simulink model "CLA_Sample"  (R2022b)
settings: Solver=FixedStepAuto  StartTime=0.0  StopTime=Inf  RelTol=1e-3  EnableMultiTasking=on
model workspace (MAT data in the model file):
  ADC_Gain = 1241.21212121
  DAC_Gain = 0.000805860805861
  Inductor_Current_Divider_Gain_Phase_A = 33.4
  Inductor_Current_Divider_Gain_Phase_B = 33.4
  Vbulk_Divider_Gain = 276.854928018
  Vin_Divider_Gain = 556.17352614
undefined symbols (not defined in the file or in its folder): GPTRIP1SEL, GPTRIP2SEL, SCI_A_Transmit, SCI_A_Transmit_Current_Suffix, SCI_A_Transmit_one_shot_Suffix, SCI_A_Transmit_Polarity_Suffix, SCI_A_Transmit_relay_Suffix, SCI_A_Transmit_Vbulk_Suffix, SCI_A_Transmit_Vin_rms_Suffix, SCI_A_Transmit_Vin_Suffix, SCI_A_Transmit_Vmid_Suffix, SCI_A_Transmit_Vp_Suffix, SCI_A_Transmit_Vpfc_Suffix, TZ1, TZ2
libraries: c280xlib x33, simulink x17, c2802xlib x15, c2000lib x1, c2806xlib x1
(part 2 of 5)

== system CLA_Sample/Calibration,RMS, Fault Protection @5kHz/Relay control ==
  note: 0.2 x ms
  note: This block will be executed at every 1 mili second. (1kHz)
  function : TriggerPort  TriggerType=function-call  VariantControl=(inherit)
  ADC Gain : Subsystem
  Data Store Memory1 : DataStoreMemory  DataStoreName=RELAY_START_DELAY  WriteAfterWriteMsg=warning  ShowAdditionalParam=off
  Data Store Read1 : DataStoreRead  DataStoreName=RELAY_START_DELAY  IndexOptions=Index vector (dialog)  Indices=1  OutputSizes=1
  Data Store Read3 : DataStoreRead  DataStoreName=Vin_peak_ADC_Phase_A  IndexOptions=Index vector (dialog)  Indices=1  OutputSizes=1
  Data Store Read4 : DataStoreRead  DataStoreName=Relay_TurnON_Threshold  IndexOptions=Index vector (dialog)  Indices=1  OutputSizes=1
  Data Store Read5 : DataStoreRead  DataStoreName=PFC_en  IndexOptions=Index vector (dialog)  Indices=1  OutputSizes=1
  Data Store Write1 : DataStoreWrite  DataStoreName=RELAY_START_DELAY  IndexOptions=Index vector (dialog)  Indices=1  OutputSizes=1
  Data Store Write6 : DataStoreWrite  DataStoreName=Relay_started  IndexOptions=Index vector (dialog)  Indices=1  OutputSizes=1
  Relay_Control : Stateflow chart  TreatAsAtomicUnit=on
  Relay_GPIO1 : c280xlib/Digital Output  GPIO_Number=GPIO8~GPIO15  GPIO_Bit0=on  GPIO_BIT0_Toggle=off  GPIO_Bit1=off  GPIO_BIT1_Toggle=off  GPIO_Bit2=off  GPIO_BIT2_Toggle=off  GPIO_Bit3=off  GPIO_BIT3_Toggle=off  GPIO_Bit4=off  GPIO_BIT4_Toggle=off  GPIO_Bit5=off  GPIO_BIT5_Toggle=off  GPIO_Bit6=off  GPIO_BIT6_Toggle=off  GPIO_Bit7=off  GPIO_BIT7_Toggle=off
  Subsystem : Subsystem  Commented=on
  ms : Constant  Value=150
  wires:
  ADC Gain/1(Out1) -> Relay_Control/2(Relay_TurnON_Threshold_ADC)
  Data Store Read5/1 -> Relay_Control/4(PFC_en)
  ms/1 -> Data Store Write1/1
  Relay_Control/2(PWM_Turned_on) -> Data Store Write6/1
  Data Store Read4/1 -> ADC Gain/1(In1)
  Relay_Control/1(Relay_Started) -> Relay_GPIO1/1
  Data Store Read1/1 -> Relay_Control/3(RELAY_START_DELAY)
  Data Store Read3/1 -> Relay_Control/1(Vin_peak_ADC)

== system CLA_Sample/Calibration,RMS, Fault Protection @5kHz/Soft Start ==
  note: This will be used for control computation.
  function : TriggerPort  TriggerType=function-call  VariantControl=(inherit)
  Chart : Stateflow chart  TreatAsAtomicUnit=on
      settings: PortSchema="{\"entries\":[{\"content\":{\"sides\":[{\"content\":{\"connectorIds\":[\"In2\",\"In3\",\"In4\",\"In5\",\"In6\"]},\"type\":\"ConnectorPlacement.EquallySpacedRectSide\",\"uuid\":\"22b210d6-ceb6-4123-9311-ecfc1554a514\"},{\"content\":{\"connectorIds\":[\"Out2\",\"Out3\",\"Out4\"],\"side\":\"RIGHT\"},\"type\":\"ConnectorPlacement.EquallySpacedRectSide\",\"uuid\":\"bd71c4d7-1c84-49a9-97ae-3dc5e1ac2530\"},{\"content\":{\"connectorIds\":[\"In1\",\"Out1\"],\"side\":\"TOP\"},\"type\":\"ConnectorPlacement.EquallySpacedRectSide\",\"uuid\":\"720c9beb-f716-4abe-bf9b-a08f9ee3742e\"}]},\"type\":\"ConnectorPlacement.EquallySpacedConnector\",\"uuid\":\"ea96fba9-9c4e-4b61-9de0-918baa6c198f\"}],\"packageUris\":[\"http://schema.mathworks.com/mf0/Connector/R2020b\"],\"version\":\"1.0\"}"
  Data Store Read : DataStoreRead  DataStoreName=Relay_started  IndexOptions=Index vector (dialog)  Indices=1  OutputSizes=1
  Data Store Read1 : DataStoreRead  DataStoreName=Vbulk_ADC  IndexOptions=Index vector (dialog)  Indices=1  OutputSizes=1
  Data Store Read2 : DataStoreRead  DataStoreName=First_Pass  IndexOptions=Index vector (dialog)  Indices=1  OutputSizes=1
  Data Store Read3 : DataStoreRead  DataStoreName=Soft_Start  IndexOptions=Index vector (dialog)  Indices=1  OutputSizes=1
  Data Store Read4 : DataStoreRead  DataStoreName=Vbulk_Ref_ADC  IndexOptions=Index vector (dialog)  Indices=1  OutputSizes=1
  Data Store Read5 : DataStoreRead  DataStoreName=PFC_en  IndexOptions=Index vector (dialog)  Indices=1  OutputSizes=1
  Data Store Write : DataStoreWrite  DataStoreName=First_Pass  IndexOptions=Index vector (dialog)  Indices=1  OutputSizes=1
  Data Store Write2 : DataStoreWrite  DataStoreName=Vbulk_Ref_ADC_adjusted  IndexOptions=Index vector (dialog)  Indices=1  OutputSizes=1
  Data Store Write3 : DataStoreWrite  DataStoreName=Soft_Start  IndexOptions=Index vector (dialog)  Indices=1  OutputSizes=1
  wires:
  Data Store Read1/1 -> Chart/3(Vbulk_ADC)
  Data Store Read2/1 -> Chart/4("First_Pass ")
  Chart/2(First_Pass) -> Data Store Write/1
  Data Store Read3/1 -> Chart/5("Soft_Start ")
  Data Store Read4/1 -> Chart/6(Vbulk_Ref_ADC)
  Chart/4(Vbulk_Ref_ADC_adjusted) -> Data Store Write2/1
  Chart/3(Soft_Start) -> Data Store Write3/1
  Data Store Read5/1 -> Chart/2(PFC_en)
  Data Store Read/1 -> Chart/1(Relay_started)

== system CLA_Sample/Calibration,RMS, Fault Protection @5kHz/Voltage RMS//Averag Calculation ==
  function : TriggerPort  TriggerType=function-call  VariantControl=(inherit)
  Function-Call Generator : simulink/Ports & Subsystems/Function-Call Generator  sample_time=-1  numberOfIterations=1  DisallowWideOutput=off
  Function-Call Split : FunctionCallSplit  IconShape=distinctive  NumOutputPorts=4  OutputPortLayout=default
  Phase_A : Subsystem  TreatAsAtomicUnit=on
  Phase_B : Subsystem  TreatAsAtomicUnit=on
  Phase_C : Subsystem  TreatAsAtomicUnit=on
  Vbulk_ADC Averaging : Subsystem  TreatAsAtomicUnit=on
  wires:
  Function-Call Generator/1 -> Function-Call Split/1
  Function-Call Split/1 -> Vbulk_ADC Averaging/Trigger
  Function-Call Split/2 -> Phase_A/Trigger
  Function-Call Split/3 -> Phase_B/Trigger
  Function-Call Split/4 -> Phase_C/Trigger

== system CLA_Sample/Duty update via UART/Simulink Function ==
  note: Ascii to number
  SCI_Receive : TriggerPort  TriggerType=function-call  IsSimulinkFunction=on  FunctionName=SCI_Receive  FunctionVisibility=scoped  VariantControl=(inherit)
  Constant2 : Constant  Value=48
  Constant3 : Constant  Value=48
  Constant4 : Constant  Value=48
  Demux : Demux  Outputs=3
  Gain2 : Gain  Gain=100
  Gain3 : Gain  Gain=10
  Gain4 : Gain
  SCI Receive : c280xlib/SCI Receive  Priority=2  sciModule=A  dataHead=''  headerCheckMaxCount=16  dataTail=''  dataType=uint8  dataLenOptions=Length via dialog  dataDim=3  maxDataLength=100  initValue=0  errOption=Output custom value  errValue=0  sampleTime=-1  blockingMode=on  timeOut=0.01944  outputStatus=off
      settings: LibrarySourceBlock=c2806xlib/SCI Receive
  Sum2 : Sum  Inputs=|+-
  Sum3 : Sum  Inputs=|+-
  Sum4 : Sum  Inputs=|+-
  Sum5 : Sum  Inputs=|+++  AccumDataTypeStr=double  OutDataTypeStr=double
  y : ArgOut  DisableCoverage=on  ArgumentName=y
  wires:
  Constant4/1 -> Sum4/2
  SCI Receive/1 -> Demux/1
  Gain4/1 -> Sum5/3
  Constant2/1 -> Sum2/2
  Demux/1 -> Sum2/1
  Sum3/1 -> Gain3/1
  Demux/2 -> Sum3/1
  Demux/3 -> Sum4/1
  Sum4/1 -> Gain4/1
  Constant3/1 -> Sum3/2
  Sum2/1 -> Gain2/1
  Gain2/1 -> Sum5/1
  Gain3/1 -> Sum5/2
  Sum5/1 -> y/1

== system CLA_Sample/Initialize Function/Subsystem1 ==
  kHz : Inport
  % : Inport  Port=2
  Constant1 : Constant  Value=90E6
  Constant2 : Constant
  Divide : Product  Inputs=*/  RndMeth=Zero  SaturateOnIntegerOverflow=on
  Gain : Gain  Gain=1000
  Gain1 : Gain  Gain=1/100
  Product1 : Product
  Subtract : Sum  Inputs=+-
  Out1 : Outport
  Out2 : Outport  Port=2
  wires:
  kHz/1 -> Gain/1
  Constant1/1 -> Divide/1
  Gain/1 -> Divide/2
  Divide/1 -> Product1/1, Out1/1
  %/1 -> Gain1/1
  Constant2/1 -> Subtract/1
  Gain1/1 -> Subtract/2
  Subtract/1 -> Product1/2
  Product1/1 -> Out2/1

== system CLA_Sample/Initialize Function/Subsystem2 ==
  Hz : Inport
  Duty : Inport  Port=2
  128*14 divider : Gain  Gain=1/(128*14)
  Constant1 : Constant  Value=90E6
  Constant2 : Constant
  Divide : Product  Inputs=*/  RndMeth=Zero  SaturateOnIntegerOverflow=on
  Floor : Rounding  Operator=round
  Floor1 : Rounding  Operator=round
  Gain1 : Gain  Gain=1/100
  Product1 : Product
  Subtract : Sum  Inputs=+-
  Out1 : Outport
  Out2 : Outport  Port=2
  wires:
  Duty/1 -> Gain1/1
  Divide/1 -> Floor/1, Product1/1
  Floor1/1 -> Out2/1
  Hz/1 -> 128*14 divider/1
  128*14 divider/1 -> Divide/2
  Constant2/1 -> Subtract/1
  Gain1/1 -> Subtract/2
  Constant1/1 -> Divide/1
  Subtract/1 -> Product1/2
  Product1/1 -> Floor1/1
  Floor/1 -> Out1/1

== system CLA_Sample/Initialize Function/Subsystem3 ==
  kHz : Inport
  % : Inport  Port=2
  Constant1 : Constant  Value=90E6
  Constant2 : Constant
  Divide : Product  Inputs=*/  RndMeth=Zero  SaturateOnIntegerOverflow=on
  Gain : Gain  Gain=1000
  Gain1 : Gain  Gain=1/100
  Product1 : Product
  Subtract : Sum  Inputs=+-
  Out1 : Outport
  Out2 : Outport  Port=2
  wires:
  kHz/1 -> Gain/1
  Constant1/1 -> Divide/1
  Gain/1 -> Divide/2
  Divide/1 -> Product1/1, Out1/1
  %/1 -> Gain1/1
  Constant2/1 -> Subtract/1
  Gain1/1 -> Subtract/2
  Subtract/1 -> Product1/2
  Product1/1 -> Out2/1

== system CLA_Sample/PWM Update @65KHz/Closed loop PWM generation (Control) ==
  function : TriggerPort  TriggerType=function-call  VariantControl=(inherit)
  Data Store Read1 : DataStoreRead  DataStoreName=Relay_started  IndexOptions=Index vector (dialog)  Indices=1  OutputSizes=1
  Data Store Read7 : DataStoreRead  DataStoreName=PFC_en  IndexOptions=Index vector (dialog)  Indices=1  OutputSizes=1
  If : If  NumInputs=2  IfExpression=(u1 ==1) & (u2==1)  ShowElse=off
  If Action Subsystem : Subsystem  TreatAsAtomicUnit=on
  wires:
  Data Store Read7/1 -> If/1
  If/1 -> If Action Subsystem/Action
  Data Store Read1/1 -> If/2

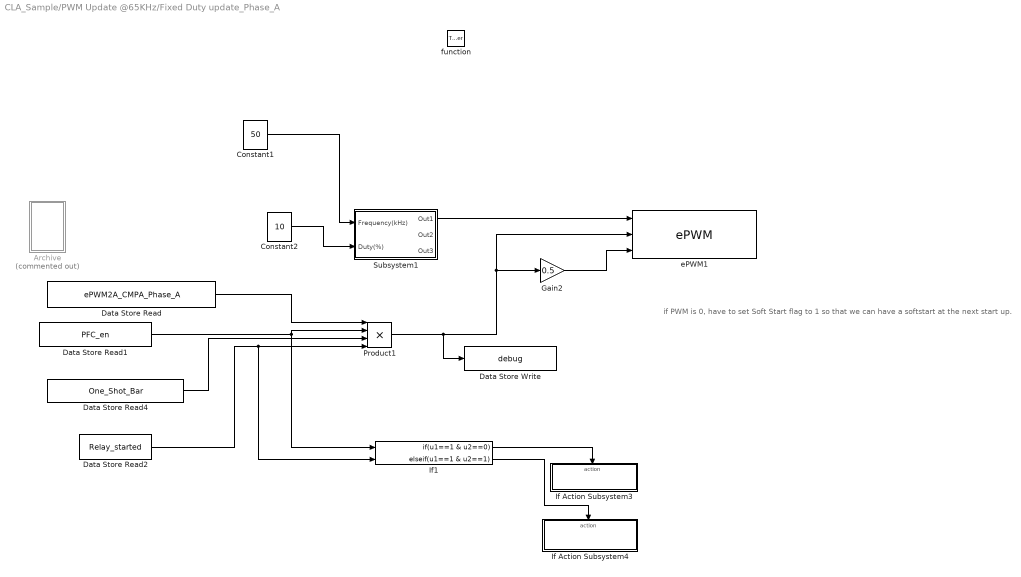
== system CLA_Sample/PWM Update @65KHz/Fixed Duty update_Phase_A ==
  note: if PWM is 0, have to set Soft Start flag to 1 so that we can have a softstart at the next start up.
  function : TriggerPort  TriggerType=function-call  VariantControl=(inherit)
  Archive : Subsystem  Commented=on
  Constant1 : Constant  Value=50
  Constant2 : Constant  Value=10
  Data Store Read : DataStoreRead  DataStoreName=ePWM2A_CMPA_Phase_A  IndexOptions=Index vector (dialog)  Indices=1  OutputSizes=1
  Data Store Read1 : DataStoreRead  DataStoreName=PFC_en  IndexOptions=Index vector (dialog)  Indices=1  OutputSizes=1
  Data Store Read2 : DataStoreRead  DataStoreName=Relay_started  IndexOptions=Index vector (dialog)  Indices=1  OutputSizes=1
  Data Store Read4 : DataStoreRead  DataStoreName=One_Shot_Bar  IndexOptions=Index vector (dialog)  Indices=1  OutputSizes=1
  Data Store Write : DataStoreWrite  DataStoreName=debug  IndexOptions=Index vector (dialog)  Indices=1  OutputSizes=1
  Gain2 : Gain  Gain=0.5
  If Action Subsystem3 : Subsystem  TreatAsAtomicUnit=on
  If Action Subsystem4 : Subsystem  TreatAsAtomicUnit=on
  If1 : If  NumInputs=2  IfExpression=u1==1 & u2==0  ElseIfExpressions=u1==1 & u2==1  ShowElse=off
  Product1 : Product  Inputs=4  OutDataTypeStr=double
  Subsystem1 : Subsystem
  ePWM1 : c2802xlib/ePWM  PwmType=C2000  useModule=ePWM2  ePWMxLINKTBPRD=Not Linked  periodUnits=Clock cycles  timerSource=Input port  timerPeriod_clk=1384  timerPeriod_sec=0.0001  tbshadow=Counter equals to zero  countingMode=Up  phaseActiveEnable=Disable  phaseDirection=Count down after sync  phaseActive=0  synchronizationEnable=off  dcaevt1Sync=off  dcbevt1Sync=off  synchronizationOption=Disable  dcbevt1SyncOut=off  dcaevt1SyncOut=off  cmpdSyncOut=off  cmpcSyncOut=off  cmpbSyncOut=off  zeroSyncOut=off  swfSyncOut=off  perSynchronizationOption=Counter equals to period (CTR=PRD)  clockPrescale=1  HSclockPrescale=1  enswap=off  ePWMxAStatus=on  ePWMxAactionLogic1=Set  ePWMxAactionLogic2=Do nothing  ePWMxAactionLogic3=Clear  ePWMxAactionLogic4=Set  ePWMxAactionLogic5=Do nothing  ePWMxAactionLogic6=Do nothing  ePWMxACSFenable=off  ePWMxACSFvalue=Forcing disable  ePWMxASFreload=Zero  ePWMxBStatus=off  ePWMxBactionLogic1=Set  ePWMxBactionLogic2=Clear  ePWMxBactionLogic3=Clear  ePWMxBactionLogic4=Do nothing  ePWMxBactionLogic5=Clear  ePWMxBactionLogic6=Set  ePWMxBCSFenable=off  ePWMxBCSFvalue=Forcing disable  ePWMxBSFreload=Zero  ePWNxBOutWay=off  ePWMxLINKCMPA=Not Linked  CMPAUnits=Clock cycles  CMPASource=Input port  CMPAValue_per=50  CMPAValue_clk=0  enCMPAshadow=Counter equals to zero (CTR=Zero)  ePWMxLINKCMPB=Not Linked  CMPBUnits=Clock cycles  CMPBSource=Input port  CMPBValue_per=50  CMPBValue_clk=0  enCMPBshadow=Counter equals to zero (CTR=Zero)  ePWMxLINKCMPC=Not Linked  CMPCUnits=Clock cycles  CMPCSource=Specify via dialog  CMPCValue_per=50  CMPCValue_clk=32000  enCMPCshadow=Counter equals to zero (CTR=Zero)  ePWMxLINKCMPD=Not Linked  CMPDUnits=Clock cycles  CMPDSource=Specify via dialog  CMPDValue_per=50  CMPDValue_clk=32000  enCMPDshadow=Counter equals to zero (CTR=Zero)  enableDBePWMxA=off  enableDBePWMxB=off  enhalfcycle=off  DBpolarity=Active high (AH)  DBedgeDelay=Positive  DBSource_ePWMxA=ePWMxA  DBSource_ePWMxB=ePWMxA  DBPeriodUnits=Clock cycles  DBperiodSource=Specify via dialog  REDperiod=0  FEDperiod=0  REDperiod_sec=0  FEDperiod_sec=0  LoadModeDBRED=Immediate without using shadow  LoadModeDBFED=Immediate without using shadow  adcstartModuleA=off  adcrequestEventA=First event  adcstartEventA=Counter is incrementing and equals to the compare B register (CTRU=CMPB)  adcstartEventA_type2=Digital Compare Module A Event 1 start of conversion (DCAEVT1.soc)  adcstartModuleB=off  adcrequestEventB=First event  adcstartEventB=Counter equals to zero (CTR=Zero)  adcstartEventB_type2=Counter equals to zero (CTR=Zero)  intEn=off  intPrd=First event  intSel=Counter equals to zero (CTR=Zero)  intSel_type2=Counter equals to zero (CTR=Zero)  hrpe=off  enHRPWM=off  HRPWM_LoadMode=Counter equals to period (CTR=PRD)  HRPWM_CTLMode=Duty or Period control mode  HRPWM_EDGMode=Both edge  hrpeb=off  enHRPWMB=off  HRPWM_LoadModeB=Counter equals to zero (CTR=ZERO)  HRPWM_CTLModeB=Duty or Period control mode  HRPWM_EDGModeB=Both edge  enHRDBRED=off  enHRDBFED=off  enSFO=on  enautoconv=on  chopperEnable=off  chopperFrequency=1  chopperFirstwidth=1  chopperDuty=12.5%  tripZonesource=Specify via dialog  tzselOSHT1=off  tzselOSHT2=off  tzselOSHT3=off  tzselOSHDCAEV1=off  tzselOSHDCBEV1=off  tzselCBC1=off  tzselCBC2=off  tzselCBC3=off  tzselCBCDCAEV2=off  tzselCBCDCBEV2=off  tzselOSHT4=off  tzselOSHT5=off  tzselOSHT6=off  tzselCBC4=off  tzselCBC5=off  tzselCBC6=off  enTzOstIntr=off  enTzCbcIntr=off  enTzDCAEVT1Intr=off  enTzDCAEVT2Intr=off  enTzDCBEVT1Intr=off  enTzDCBEVT2Intr=off  ePWMxAforced=No action  ePWMxBforced=No action  DCAEVT1forced=No action  DCBEVT1forced=No action  DCAEVT2forced=Low  DCBEVT2forced=No action  dcah=COMP1OUT input  dcal=Trip Zone 2 input (TZ2)  dcbh=Trip Zone 1 input (TZ1)  dcbl=Trip Zone 1 input (TZ1)  dcah_type2=GPTRIP1SEL/(TZ1)  dcal_type2=GPTRIP2SEL/(TZ2)  dcbh_type2=GPTRIP1SEL/(TZ1)  dcbl_type2=GPTRIP2SEL/(TZ2)  gendcaevt1=Event disabled  gendcaevt2=DCAH=high and DCAL=don't care  gendcbevt1=Event disabled  gendcbevt2=Event disabled  dcaevt1src=DCAEVT1 with sync  dcaevt2src=DCAEVT2 with async  dcbevt1src=DCBEVT1 with sync  dcbevt2src=DCBEVT2 with sync  pulsesel=Counter equals to zero (CTR=Zero)  blankinv=off  blankoffset=0  blankwidth=0  evsrcsel=Filtered version of DCAEVT1 (DCAEVT1FILT)  encape=off
      settings: LibrarySourceBlock=c2806xlib/ePWM
  wires:
  Data Store Read4/1 -> Product1/3
  Subsystem1/1(Out1) -> ePWM1/1
  Constant1/1 -> Subsystem1/1(Frequency(kHz))
  Gain2/1 -> ePWM1/3
  Product1/1 -> Data Store Write/1, ePWM1/2, Gain2/1
  Data Store Read/1 -> Product1/1
  If1/2 -> If Action Subsystem4/Action
  Data Store Read1/1 -> If1/1, Product1/2
  If1/1 -> If Action Subsystem3/Action
  Data Store Read2/1 -> Product1/4, If1/2
  Constant2/1 -> Subsystem1/2(Duty(%))

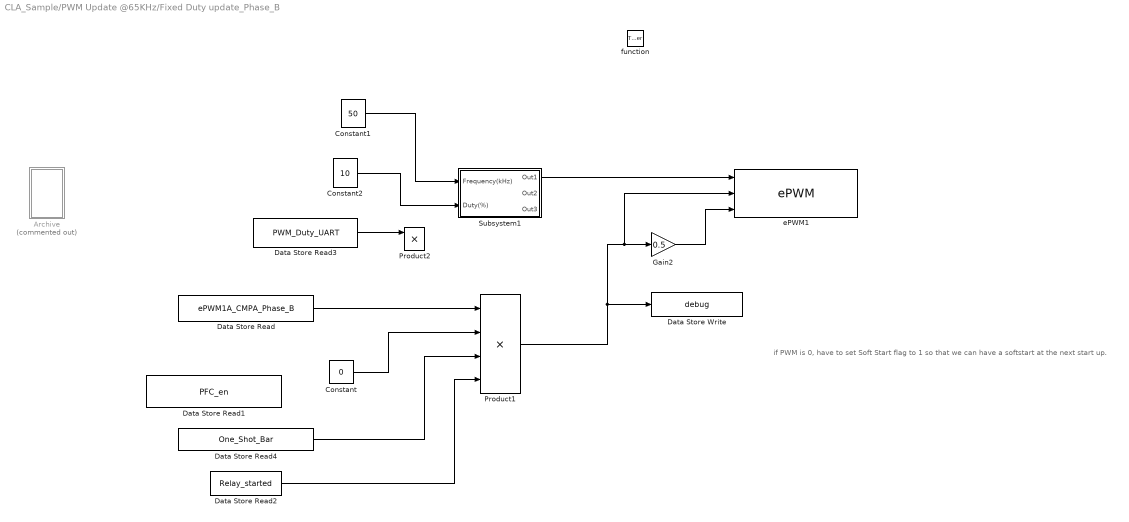
== system CLA_Sample/PWM Update @65KHz/Fixed Duty update_Phase_B ==
  note: if PWM is 0, have to set Soft Start flag to 1 so that we can have a softstart at the next start up.
  function : TriggerPort  TriggerType=function-call  VariantControl=(inherit)
  Archive : Subsystem  Commented=on
  Constant : Constant  Value=0
  Constant1 : Constant  Value=50
  Constant2 : Constant  Value=10
  Data Store Read : DataStoreRead  DataStoreName=ePWM1A_CMPA_Phase_B  IndexOptions=Index vector (dialog)  Indices=1  OutputSizes=1
  Data Store Read1 : DataStoreRead  DataStoreName=PFC_en  IndexOptions=Index vector (dialog)  Indices=1  OutputSizes=1
  Data Store Read2 : DataStoreRead  DataStoreName=Relay_started  IndexOptions=Index vector (dialog)  Indices=1  OutputSizes=1
  Data Store Read3 : DataStoreRead  DataStoreName=PWM_Duty_UART  IndexOptions=Index vector (dialog)  Indices=1  OutputSizes=1
  Data Store Read4 : DataStoreRead  DataStoreName=One_Shot_Bar  IndexOptions=Index vector (dialog)  Indices=1  OutputSizes=1
  Data Store Write : DataStoreWrite  DataStoreName=debug  IndexOptions=Index vector (dialog)  Indices=1  OutputSizes=1
  Gain2 : Gain  Gain=0.5
  Product1 : Product  Inputs=4  OutDataTypeStr=double
  Product2 : Product  OutDataTypeStr=double
  Subsystem1 : Subsystem
  ePWM1 : c2802xlib/ePWM  PwmType=C2000  useModule=ePWM1  ePWMxLINKTBPRD=Not Linked  periodUnits=Clock cycles  timerSource=Input port  timerPeriod_clk=1384  timerPeriod_sec=0.0001  tbshadow=Counter equals to zero  countingMode=Up  phaseActiveEnable=Disable  phaseDirection=Count down after sync  phaseActive=0  synchronizationEnable=off  dcaevt1Sync=off  dcbevt1Sync=off  synchronizationOption=Disable  dcbevt1SyncOut=off  dcaevt1SyncOut=off  cmpdSyncOut=off  cmpcSyncOut=off  cmpbSyncOut=off  zeroSyncOut=off  swfSyncOut=off  perSynchronizationOption=Counter equals to period (CTR=PRD)  clockPrescale=1  HSclockPrescale=1  enswap=off  ePWMxAStatus=on  ePWMxAactionLogic1=Set  ePWMxAactionLogic2=Do nothing  ePWMxAactionLogic3=Clear  ePWMxAactionLogic4=Set  ePWMxAactionLogic5=Do nothing  ePWMxAactionLogic6=Do nothing  ePWMxACSFenable=off  ePWMxACSFvalue=Forcing disable  ePWMxASFreload=Zero  ePWMxBStatus=off  ePWMxBactionLogic1=Set  ePWMxBactionLogic2=Clear  ePWMxBactionLogic3=Clear  ePWMxBactionLogic4=Do nothing  ePWMxBactionLogic5=Clear  ePWMxBactionLogic6=Set  ePWMxBCSFenable=off  ePWMxBCSFvalue=Forcing disable  ePWMxBSFreload=Zero  ePWNxBOutWay=off  ePWMxLINKCMPA=Not Linked  CMPAUnits=Clock cycles  CMPASource=Input port  CMPAValue_per=50  CMPAValue_clk=0  enCMPAshadow=Counter equals to zero (CTR=Zero)  ePWMxLINKCMPB=Not Linked  CMPBUnits=Clock cycles  CMPBSource=Input port  CMPBValue_per=50  CMPBValue_clk=0  enCMPBshadow=Counter equals to zero (CTR=Zero)  ePWMxLINKCMPC=Not Linked  CMPCUnits=Clock cycles  CMPCSource=Specify via dialog  CMPCValue_per=50  CMPCValue_clk=32000  enCMPCshadow=Counter equals to zero (CTR=Zero)  ePWMxLINKCMPD=Not Linked  CMPDUnits=Clock cycles  CMPDSource=Specify via dialog  CMPDValue_per=50  CMPDValue_clk=32000  enCMPDshadow=Counter equals to zero (CTR=Zero)  enableDBePWMxA=off  enableDBePWMxB=off  enhalfcycle=off  DBpolarity=Active high (AH)  DBedgeDelay=Positive  DBSource_ePWMxA=ePWMxA  DBSource_ePWMxB=ePWMxA  DBPeriodUnits=Clock cycles  DBperiodSource=Specify via dialog  REDperiod=0  FEDperiod=0  REDperiod_sec=0  FEDperiod_sec=0  LoadModeDBRED=Immediate without using shadow  LoadModeDBFED=Immediate without using shadow  adcstartModuleA=on  adcrequestEventA=First event  adcstartEventA=Counter is incrementing and equals to the compare B register (CTRU=CMPB)  adcstartEventA_type2=Digital Compare Module A Event 1 start of conversion (DCAEVT1.soc)  adcstartModuleB=off  adcrequestEventB=First event  adcstartEventB=Counter equals to zero (CTR=Zero)  adcstartEventB_type2=Counter equals to zero (CTR=Zero)  intEn=on  intPrd=First event  intSel=Counter equals to zero (CTR=Zero)  intSel_type2=Counter equals to zero (CTR=Zero)  hrpe=off  enHRPWM=off  HRPWM_LoadMode=Counter equals to period (CTR=PRD)  HRPWM_CTLMode=Duty or Period control mode  HRPWM_EDGMode=Both edge  hrpeb=off  enHRPWMB=off  HRPWM_LoadModeB=Counter equals to zero (CTR=ZERO)  HRPWM_CTLModeB=Duty or Period control mode  HRPWM_EDGModeB=Both edge  enHRDBRED=off  enHRDBFED=off  enSFO=on  enautoconv=on  chopperEnable=off  chopperFrequency=1  chopperFirstwidth=1  chopperDuty=12.5%  tripZonesource=Specify via dialog  tzselOSHT1=off  tzselOSHT2=off  tzselOSHT3=off  tzselOSHDCAEV1=off  tzselOSHDCBEV1=off  tzselCBC1=off  tzselCBC2=off  tzselCBC3=off  tzselCBCDCAEV2=off  tzselCBCDCBEV2=off  tzselOSHT4=off  tzselOSHT5=off  tzselOSHT6=off  tzselCBC4=off  tzselCBC5=off  tzselCBC6=off  enTzOstIntr=off  enTzCbcIntr=off  enTzDCAEVT1Intr=off  enTzDCAEVT2Intr=off  enTzDCBEVT1Intr=off  enTzDCBEVT2Intr=off  ePWMxAforced=No action  ePWMxBforced=No action  DCAEVT1forced=No action  DCBEVT1forced=No action  DCAEVT2forced=No action  DCBEVT2forced=No action  dcah=Trip Zone 2 input (TZ2)  dcal=Trip Zone 2 input (TZ2)  dcbh=Trip Zone 1 input (TZ1)  dcbl=Trip Zone 1 input (TZ1)  dcah_type2=GPTRIP1SEL/(TZ1)  dcal_type2=GPTRIP2SEL/(TZ2)  dcbh_type2=GPTRIP1SEL/(TZ1)  dcbl_type2=GPTRIP2SEL/(TZ2)  gendcaevt1=Event disabled  gendcaevt2=Event disabled  gendcbevt1=Event disabled  gendcbevt2=Event disabled  dcaevt1src=DCAEVT1 with sync  dcaevt2src=DCAEVT2 with sync  dcbevt1src=DCBEVT1 with sync  dcbevt2src=DCBEVT2 with sync  pulsesel=Counter equals to zero (CTR=Zero)  blankinv=off  blankoffset=0  blankwidth=0  evsrcsel=Filtered version of DCAEVT1 (DCAEVT1FILT)  encape=off
      settings: LibrarySourceBlock=c2806xlib/ePWM
  wires:
  Subsystem1/1(Out1) -> ePWM1/1
  Constant1/1 -> Subsystem1/1(Frequency(kHz))
  Product1/1 -> ePWM1/2, Gain2/1, Data Store Write/1
  Data Store Read/1 -> Product1/1
  Data Store Read4/1 -> Product1/3
  Data Store Read2/1 -> Product1/4
  Data Store Read3/1 -> Product2/1
  Constant2/1 -> Subsystem1/2(Duty(%))
  Gain2/1 -> ePWM1/3
  Constant/1 -> Product1/2

== system CLA_Sample/PWM Update @65KHz/Fixed Duty update_Phase_C ==
  note: if PWM is 0, have to set Soft Start flag to 1 so that we can have a softstart at the next start up.
  function : TriggerPort  TriggerType=function-call  VariantControl=(inherit)
  Archive : Subsystem  Commented=on
  Constant1 : Constant  Value=50
  Constant2 : Constant  Value=10
  Data Store Read : DataStoreRead  DataStoreName=ePWM3A_CMPA_Phase_C  IndexOptions=Index vector (dialog)  Indices=1  OutputSizes=1
  Data Store Read1 : DataStoreRead  DataStoreName=PFC_en  IndexOptions=Index vector (dialog)  Indices=1  OutputSizes=1
  Data Store Read2 : DataStoreRead  DataStoreName=Relay_started  IndexOptions=Index vector (dialog)  Indices=1  OutputSizes=1
  Data Store Read4 : DataStoreRead  DataStoreName=One_Shot_Bar  IndexOptions=Index vector (dialog)  Indices=1  OutputSizes=1
  Data Store Write : DataStoreWrite  DataStoreName=debug  IndexOptions=Index vector (dialog)  Indices=1  OutputSizes=1
  Gain2 : Gain  Gain=0.5
  Product1 : Product  Inputs=4  OutDataTypeStr=double
  Subsystem1 : Subsystem
  ePWM1 : c2802xlib/ePWM  PwmType=C2000  useModule=ePWM3  ePWMxLINKTBPRD=Not Linked  periodUnits=Clock cycles  timerSource=Input port  timerPeriod_clk=1384  timerPeriod_sec=0.0001  tbshadow=Counter equals to zero  countingMode=Up  phaseActiveEnable=Disable  phaseDirection=Count down after sync  phaseActive=0  synchronizationEnable=off  dcaevt1Sync=off  dcbevt1Sync=off  synchronizationOption=Disable  dcbevt1SyncOut=off  dcaevt1SyncOut=off  cmpdSyncOut=off  cmpcSyncOut=off  cmpbSyncOut=off  zeroSyncOut=off  swfSyncOut=off  perSynchronizationOption=Counter equals to period (CTR=PRD)  clockPrescale=1  HSclockPrescale=1  enswap=off  ePWMxAStatus=on  ePWMxAactionLogic1=Set  ePWMxAactionLogic2=Do nothing  ePWMxAactionLogic3=Clear  ePWMxAactionLogic4=Set  ePWMxAactionLogic5=Do nothing  ePWMxAactionLogic6=Do nothing  ePWMxACSFenable=off  ePWMxACSFvalue=Forcing disable  ePWMxASFreload=Zero  ePWMxBStatus=off  ePWMxBactionLogic1=Set  ePWMxBactionLogic2=Clear  ePWMxBactionLogic3=Clear  ePWMxBactionLogic4=Do nothing  ePWMxBactionLogic5=Clear  ePWMxBactionLogic6=Set  ePWMxBCSFenable=off  ePWMxBCSFvalue=Forcing disable  ePWMxBSFreload=Zero  ePWNxBOutWay=off  ePWMxLINKCMPA=Not Linked  CMPAUnits=Clock cycles  CMPASource=Input port  CMPAValue_per=50  CMPAValue_clk=0  enCMPAshadow=Counter equals to zero (CTR=Zero)  ePWMxLINKCMPB=Not Linked  CMPBUnits=Clock cycles  CMPBSource=Input port  CMPBValue_per=50  CMPBValue_clk=0  enCMPBshadow=Counter equals to zero (CTR=Zero)  ePWMxLINKCMPC=Not Linked  CMPCUnits=Clock cycles  CMPCSource=Specify via dialog  CMPCValue_per=50  CMPCValue_clk=32000  enCMPCshadow=Counter equals to zero (CTR=Zero)  ePWMxLINKCMPD=Not Linked  CMPDUnits=Clock cycles  CMPDSource=Specify via dialog  CMPDValue_per=50  CMPDValue_clk=32000  enCMPDshadow=Counter equals to zero (CTR=Zero)  enableDBePWMxA=off  enableDBePWMxB=off  enhalfcycle=off  DBpolarity=Active high (AH)  DBedgeDelay=Positive  DBSource_ePWMxA=ePWMxA  DBSource_ePWMxB=ePWMxA  DBPeriodUnits=Clock cycles  DBperiodSource=Specify via dialog  REDperiod=0  FEDperiod=0  REDperiod_sec=0  FEDperiod_sec=0  LoadModeDBRED=Immediate without using shadow  LoadModeDBFED=Immediate without using shadow  adcstartModuleA=off  adcrequestEventA=First event  adcstartEventA=Counter is incrementing and equals to the compare B register (CTRU=CMPB)  adcstartEventA_type2=Digital Compare Module A Event 1 start of conversion (DCAEVT1.soc)  adcstartModuleB=off  adcrequestEventB=First event  adcstartEventB=Counter equals to zero (CTR=Zero)  adcstartEventB_type2=Counter equals to zero (CTR=Zero)  intEn=off  intPrd=First event  intSel=Counter equals to zero (CTR=Zero)  intSel_type2=Counter equals to zero (CTR=Zero)  hrpe=off  enHRPWM=off  HRPWM_LoadMode=Counter equals to period (CTR=PRD)  HRPWM_CTLMode=Duty or Period control mode  HRPWM_EDGMode=Both edge  hrpeb=off  enHRPWMB=off  HRPWM_LoadModeB=Counter equals to zero (CTR=ZERO)  HRPWM_CTLModeB=Duty or Period control mode  HRPWM_EDGModeB=Both edge  enHRDBRED=off  enHRDBFED=off  enSFO=on  enautoconv=on  chopperEnable=off  chopperFrequency=1  chopperFirstwidth=1  chopperDuty=12.5%  tripZonesource=Specify via dialog  tzselOSHT1=off  tzselOSHT2=off  tzselOSHT3=off  tzselOSHDCAEV1=off  tzselOSHDCBEV1=off  tzselCBC1=off  tzselCBC2=off  tzselCBC3=off  tzselCBCDCAEV2=off  tzselCBCDCBEV2=off  tzselOSHT4=off  tzselOSHT5=off  tzselOSHT6=off  tzselCBC4=off  tzselCBC5=off  tzselCBC6=off  enTzOstIntr=off  enTzCbcIntr=off  enTzDCAEVT1Intr=off  enTzDCAEVT2Intr=off  enTzDCBEVT1Intr=off  enTzDCBEVT2Intr=off  ePWMxAforced=No action  ePWMxBforced=No action  DCAEVT1forced=No action  DCBEVT1forced=No action  DCAEVT2forced=No action  DCBEVT2forced=No action  dcah=Trip Zone 2 input (TZ2)  dcal=Trip Zone 2 input (TZ2)  dcbh=Trip Zone 1 input (TZ1)  dcbl=Trip Zone 1 input (TZ1)  dcah_type2=GPTRIP1SEL/(TZ1)  dcal_type2=GPTRIP2SEL/(TZ2)  dcbh_type2=GPTRIP1SEL/(TZ1)  dcbl_type2=GPTRIP2SEL/(TZ2)  gendcaevt1=Event disabled  gendcaevt2=Event disabled  gendcbevt1=Event disabled  gendcbevt2=Event disabled  dcaevt1src=DCAEVT1 with sync  dcaevt2src=DCAEVT2 with sync  dcbevt1src=DCBEVT1 with sync  dcbevt2src=DCBEVT2 with sync  pulsesel=Counter equals to zero (CTR=Zero)  blankinv=off  blankoffset=0  blankwidth=0  evsrcsel=Filtered version of DCAEVT1 (DCAEVT1FILT)  encape=off
      settings: LibrarySourceBlock=c2806xlib/ePWM
  wires:
  Subsystem1/1(Out1) -> ePWM1/1
  Constant1/1 -> Subsystem1/1(Frequency(kHz))
  Product1/1 -> ePWM1/2, Gain2/1, Data Store Write/1
  Data Store Read/1 -> Product1/1
  Data Store Read1/1 -> Product1/2
  Data Store Read4/1 -> Product1/3
  Data Store Read2/1 -> Product1/4
  Constant2/1 -> Subsystem1/2(Duty(%))
  Gain2/1 -> ePWM1/3

== system CLA_Sample/UART reporting @ 1Hz/Data_calculation ==
  function : TriggerPort  TriggerType=function-call  VariantControl=(inherit)
  DataCalculation_Phase_A : Subsystem  TreatAsAtomicUnit=on
  DataCalculation_Phase_B : Subsystem  TreatAsAtomicUnit=on
  DataCalculation_Phase_C : Subsystem  TreatAsAtomicUnit=on
  Function-Call Generator : simulink/Ports & Subsystems/Function-Call Generator  sample_time=-1  numberOfIterations=1  DisallowWideOutput=off
  Function-Call Split : FunctionCallSplit  IconShape=distinctive  NumOutputPorts=4  OutputPortLayout=default
  Vbulk&Vmid : Subsystem  TreatAsAtomicUnit=on
  wires:
  Function-Call Generator/1 -> Function-Call Split/1
  Function-Call Split/1 -> DataCalculation_Phase_A/Trigger
  Function-Call Split/2 -> DataCalculation_Phase_B/Trigger
  Function-Call Split/3 -> DataCalculation_Phase_C/Trigger
  Function-Call Split/4 -> Vbulk&Vmid/Trigger

== system CLA_Sample/UART reporting @ 1Hz/Phase_A ==
  function : TriggerPort  TriggerType=function-call  VariantControl=(inherit)
  Duty_control_loop_Phase_A : Subsystem  Commented=on  TreatAsAtomicUnit=on
  Function-Call Generator : simulink/Ports & Subsystems/Function-Call Generator  sample_time=-1  numberOfIterations=1  DisallowWideOutput=off
  Function-Call Split : FunctionCallSplit  IconShape=distinctive  NumOutputPorts=5  OutputPortLayout=default
  Send Inductor_Current (A) : Subsystem  TreatAsAtomicUnit=on
  Send PFC_en_Phase_A : Subsystem  Commented=on  TreatAsAtomicUnit=on
  Send Vin (V) : Subsystem  Commented=on  TreatAsAtomicUnit=on
  Send Vin_rms (V) : Subsystem  TreatAsAtomicUnit=on
  wires:
  Function-Call Generator/1 -> Function-Call Split/1
  Function-Call Split/1 -> Send Vin (V)/Trigger
  Function-Call Split/2 -> Send Inductor_Current (A)/Trigger
  Function-Call Split/3 -> Send Vin_rms (V)/Trigger
  Function-Call Split/4 -> Send PFC_en_Phase_A/Trigger
  Function-Call Split/5 -> Duty_control_loop_Phase_A/Trigger

== system CLA_Sample/UART reporting @ 1Hz/Phase_B ==
  function : TriggerPort  TriggerType=function-call  VariantControl=(inherit)
  Duty_control_loop_Phase_B : Subsystem  Commented=on  TreatAsAtomicUnit=on
  Function-Call Generator : simulink/Ports & Subsystems/Function-Call Generator  sample_time=-1  numberOfIterations=1  DisallowWideOutput=off
  Function-Call Split : FunctionCallSplit  IconShape=distinctive  NumOutputPorts=5  OutputPortLayout=default
  Send Inductor_Current (A) : Subsystem  TreatAsAtomicUnit=on
  Send PFC_en_Phase_B : Subsystem  Commented=on  TreatAsAtomicUnit=on
  Send Vin (V) : Subsystem  Commented=on  TreatAsAtomicUnit=on
  Send Vin_rms (V) : Subsystem  TreatAsAtomicUnit=on
  wires:
  Function-Call Generator/1 -> Function-Call Split/1
  Function-Call Split/1 -> Send Vin (V)/Trigger
  Function-Call Split/2 -> Send Inductor_Current (A)/Trigger
  Function-Call Split/3 -> Send Vin_rms (V)/Trigger
  Function-Call Split/4 -> Send PFC_en_Phase_B/Trigger
  Function-Call Split/5 -> Duty_control_loop_Phase_B/Trigger

== system CLA_Sample/UART reporting @ 1Hz/Phase_C ==
  function : TriggerPort  TriggerType=function-call  VariantControl=(inherit)
  Duty_control_loop_Phase_C : Subsystem  Commented=on  TreatAsAtomicUnit=on
  Function-Call Generator : simulink/Ports & Subsystems/Function-Call Generator  sample_time=-1  numberOfIterations=1  DisallowWideOutput=off
  Function-Call Split : FunctionCallSplit  IconShape=distinctive  NumOutputPorts=5  OutputPortLayout=default
  Send Inductor_Current (A) : Subsystem  TreatAsAtomicUnit=on
  Send PFC_en_Phase_C : Subsystem  Commented=on  TreatAsAtomicUnit=on
  Send Vin (V) : Subsystem  Commented=on  TreatAsAtomicUnit=on
  Send Vin_rms (V) : Subsystem  TreatAsAtomicUnit=on
  wires:
  Function-Call Generator/1 -> Function-Call Split/1
  Function-Call Split/1 -> Send Vin (V)/Trigger
  Function-Call Split/2 -> Send Inductor_Current (A)/Trigger
  Function-Call Split/3 -> Send Vin_rms (V)/Trigger
  Function-Call Split/4 -> Send PFC_en_Phase_C/Trigger
  Function-Call Split/5 -> Duty_control_loop_Phase_C/Trigger

== system CLA_Sample/UART reporting @ 1Hz/SCI_A_Transmit_function ==
  SCI_A_Transmit : TriggerPort  TriggerType=function-call  IsSimulinkFunction=on  FunctionName=SCI_A_Transmit  FunctionVisibility=scoped  VariantControl=(inherit)
  Add Constant{,1..4} (5 alike) : Bias  Bias=48  SaturateOnIntegerOverflow=off
  Constant : Constant  Value=10000
  MATLAB Function : MATLAB Function  TreatAsAtomicUnit=on
  Mux : Mux  Inputs=5
  SCI Transmit : c280xlib/SCI Transmit  sciModule=A  dataHead=''  dataTail=''  blockingMode=on  outputStatus=off
  u : ArgIn  DisableCoverage=on  ArgumentName=u
  wires:
  Mux/1 -> SCI Transmit/1
  Add Constant4/1 -> Mux/5
  Add Constant3/1 -> Mux/4
  Add Constant2/1 -> Mux/3
  Add Constant1/1 -> Mux/2
  Add Constant/1 -> Mux/1
  MATLAB Function/1(Digit_5) -> Add Constant/1
  MATLAB Function/2(Digit_4) -> Add Constant1/1
  MATLAB Function/3(Digit_3) -> Add Constant2/1
  MATLAB Function/4(Digit_2) -> Add Constant3/1
  MATLAB Function/5(Digit_1) -> Add Constant4/1
  Constant/1 -> MATLAB Function/2(Divider)
  u/1 -> MATLAB Function/1(Main_number)

== system CLA_Sample/UART reporting @ 1Hz/SCI_A_Transmit_function1 ==
  note: 86 Decimal = 'V' in ASCII
  SCI_A_Transmit_Vbulk_Suffix : TriggerPort  TriggerType=function-call  IsSimulinkFunction=on  FunctionName=SCI_A_Transmit_Vbulk_Suffix  FunctionVisibility=scoped  VariantControl=(inherit)
  SCI Transmit : c280xlib/SCI Transmit  sciModule=A  dataHead=''  dataTail=10  blockingMode=on  outputStatus=off
  Vbulk : Constant  Value=[86 98 117 108 107]  OutDataTypeStr=uint8
  wires:
  Vbulk/1 -> SCI Transmit/1

== system CLA_Sample/UART reporting @ 1Hz/SCI_A_Transmit_function10 ==
  SCI_A_Transmit_one_shot_Suffix : TriggerPort  TriggerType=function-call  IsSimulinkFunction=on  FunctionName=SCI_A_Transmit_relay_Suffix  FunctionVisibility=scoped  VariantControl=(inherit)
  P O L : Constant  Value=[82 69 76]  OutDataTypeStr=uint8
  SCI Transmit : c280xlib/SCI Transmit  sciModule=A  dataHead=''  dataTail=10  blockingMode=on  outputStatus=off
  wires:
  P O L/1 -> SCI Transmit/1

== system CLA_Sample/UART reporting @ 1Hz/SCI_A_Transmit_function2 ==
  note: 65 Decimal = 'A' in ASCII
  SCI_A_Transmit_Current_Suffix : TriggerPort  TriggerType=function-call  IsSimulinkFunction=on  FunctionName=SCI_A_Transmit_Current_Suffix  FunctionVisibility=scoped  VariantControl=(inherit)
  Current : Constant  Value=[65]  OutDataTypeStr=uint8
  SCI Transmit : c280xlib/SCI Transmit  sciModule=A  dataHead=''  dataTail=10  blockingMode=on  outputStatus=off
  wires:
  Current/1 -> SCI Transmit/1

== system CLA_Sample/UART reporting @ 1Hz/SCI_A_Transmit_function3 ==
  note: 86 Decimal = 'V' in ASCII
  SCI_A_Transmit_Vin_Suffix : TriggerPort  TriggerType=function-call  IsSimulinkFunction=on  FunctionName=SCI_A_Transmit_Vin_Suffix  FunctionVisibility=scoped  VariantControl=(inherit)
  SCI Transmit : c280xlib/SCI Transmit  sciModule=A  dataHead=''  dataTail=10  blockingMode=on  outputStatus=off
  Vin : Constant  Value=[86 105 110]  OutDataTypeStr=uint8
  wires:
  Vin/1 -> SCI Transmit/1

== system CLA_Sample/UART reporting @ 1Hz/SCI_A_Transmit_function4 ==
  note: 86 Decimal = 'V' in ASCII
  SCI_A_Transmit_Vin_rms_Suffix : TriggerPort  TriggerType=function-call  IsSimulinkFunction=on  FunctionName=SCI_A_Transmit_Vin_rms_Suffix  FunctionVisibility=scoped  VariantControl=(inherit)
  SCI Transmit : c280xlib/SCI Transmit  sciModule=A  dataHead=''  dataTail=10  blockingMode=on  outputStatus=off
  Vrms : Constant  Value=[86 114 109 115]  OutDataTypeStr=uint8
  wires:
  Vrms/1 -> SCI Transmit/1

== system CLA_Sample/UART reporting @ 1Hz/SCI_A_Transmit_function5 ==
  SCI_A_Transmit_Polarity_Suffix : TriggerPort  TriggerType=function-call  IsSimulinkFunction=on  FunctionName=SCI_A_Transmit_Polarity_Suffix  FunctionVisibility=scoped  VariantControl=(inherit)
  P O L : Constant  Value=[80 79 76]  OutDataTypeStr=uint8
  SCI Transmit : c280xlib/SCI Transmit  sciModule=A  dataHead=''  dataTail=10  blockingMode=on  outputStatus=off
  wires:
  P O L/1 -> SCI Transmit/1

== system CLA_Sample/UART reporting @ 1Hz/SCI_A_Transmit_function6 ==
  SCI_A_Transmit_Vp_Suffix : TriggerPort  TriggerType=function-call  IsSimulinkFunction=on  FunctionName=SCI_A_Transmit_Vp_Suffix  FunctionVisibility=scoped  VariantControl=(inherit)
  SCI Transmit : c280xlib/SCI Transmit  sciModule=A  dataHead=''  dataTail=10  blockingMode=on  outputStatus=off
  "VP " : Constant  Value=[86 80]  OutDataTypeStr=uint8
  wires:
  "VP "/1 -> SCI Transmit/1

== system CLA_Sample/UART reporting @ 1Hz/SCI_A_Transmit_function7 ==
  note: 86 Decimal = 'V' in ASCII
  SCI_A_Transmit_Vmid_Suffix : TriggerPort  TriggerType=function-call  IsSimulinkFunction=on  FunctionName=SCI_A_Transmit_Vmid_Suffix  FunctionVisibility=scoped  VariantControl=(inherit)
  SCI Transmit : c280xlib/SCI Transmit  sciModule=A  dataHead=''  dataTail=10  blockingMode=on  outputStatus=off
  Vmid : Constant  Value=[86 109 105 100]  OutDataTypeStr=uint8
  wires:
  Vmid/1 -> SCI Transmit/1

== system CLA_Sample/UART reporting @ 1Hz/SCI_A_Transmit_function8 ==
  SCI_A_Transmit_Vpfc_Suffix : TriggerPort  TriggerType=function-call  IsSimulinkFunction=on  FunctionName=SCI_A_Transmit_Vpfc_Suffix  FunctionVisibility=scoped  VariantControl=(inherit)
  SCI Transmit : c280xlib/SCI Transmit  sciModule=A  dataHead=''  dataTail=10  blockingMode=on  outputStatus=off
  "VPFC " : Constant  Value=[86 80 70 67]  OutDataTypeStr=uint8
  wires:
  "VPFC "/1 -> SCI Transmit/1

== system CLA_Sample/UART reporting @ 1Hz/SCI_A_Transmit_function9 ==
  SCI_A_Transmit_one_shot_Suffix : TriggerPort  TriggerType=function-call  IsSimulinkFunction=on  FunctionName=SCI_A_Transmit_one_shot_Suffix  FunctionVisibility=scoped  VariantControl=(inherit)
  P O L : Constant  Value=[79 78 69]  OutDataTypeStr=uint8
  SCI Transmit : c280xlib/SCI Transmit  sciModule=A  dataHead=''  dataTail=10  blockingMode=on  outputStatus=off
  wires:
  P O L/1 -> SCI Transmit/1

== system CLA_Sample/UART reporting @ 1Hz/Send PFC_en ==
  function : TriggerPort  TriggerType=function-call  VariantControl=(inherit)
  Data Store Read : DataStoreRead  DataStoreName=PFC_en  IndexOptions=Index vector (dialog)  Indices=1  OutputSizes=1
  Function Caller1 : FunctionCaller  FunctionPrototype=SCI_A_Transmit(u)  InputArgumentSpecifications=<Enter example>  OutputArgumentSpecifications=<Enter example>
  Function Caller2 : FunctionCaller  FunctionPrototype=SCI_A_Transmit_Vpfc_Suffix()  InputArgumentSpecifications=<Enter example>  OutputArgumentSpecifications=<Enter example>
  wires:
  Data Store Read/1 -> Function Caller1/1

== system CLA_Sample/UART reporting @ 1Hz/Send Relay_started ==
  function : TriggerPort  TriggerType=function-call  VariantControl=(inherit)
  Data Store Read : DataStoreRead  DataStoreName=Relay_started  IndexOptions=Index vector (dialog)  Indices=1  OutputSizes=1
  Function Caller1 : FunctionCaller  FunctionPrototype=SCI_A_Transmit(u)  InputArgumentSpecifications=<Enter example>  OutputArgumentSpecifications=<Enter example>
  Function Caller2 : FunctionCaller  FunctionPrototype=SCI_A_Transmit_relay_Suffix()  InputArgumentSpecifications=<Enter example>  OutputArgumentSpecifications=<Enter example>
  wires:
  Data Store Read/1 -> Function Caller1/1

== system CLA_Sample/UART reporting @ 1Hz/Send Vbulk (V) ==
  function : TriggerPort  TriggerType=function-call  VariantControl=(inherit)
  Data Store Read : DataStoreRead  DataStoreName=Vbulk  IndexOptions=Index vector (dialog)  Indices=1  OutputSizes=1
  Function Caller1 : FunctionCaller  FunctionPrototype=SCI_A_Transmit(u)  InputArgumentSpecifications=<Enter example>  OutputArgumentSpecifications=<Enter example>
  Function Caller2 : FunctionCaller  FunctionPrototype=SCI_A_Transmit_Vbulk_Suffix()  InputArgumentSpecifications=<Enter example>  OutputArgumentSpecifications=<Enter example>
  wires:
  Data Store Read/1 -> Function Caller1/1

== system CLA_Sample/UART reporting @ 1Hz/Send Vmid ==
  function : TriggerPort  TriggerType=function-call  VariantControl=(inherit)
  Data Store Read : DataStoreRead  DataStoreName=Vmid  IndexOptions=Index vector (dialog)  Indices=1  OutputSizes=1
  Function Caller1 : FunctionCaller  FunctionPrototype=SCI_A_Transmit(u)  InputArgumentSpecifications=<Enter example>  OutputArgumentSpecifications=<Enter example>
  Function Caller2 : FunctionCaller  FunctionPrototype=SCI_A_Transmit_Vmid_Suffix()  InputArgumentSpecifications=<Enter example>  OutputArgumentSpecifications=<Enter example>
  wires:
  Data Store Read/1 -> Function Caller1/1

== system CLA_Sample/UART reporting @ 1Hz/Send one_shot_bar ==
  function : TriggerPort  TriggerType=function-call  VariantControl=(inherit)
  Data Store Read : DataStoreRead  DataStoreName=One_Shot_Bar  IndexOptions=Index vector (dialog)  Indices=1  OutputSizes=1
  Function Caller1 : FunctionCaller  FunctionPrototype=SCI_A_Transmit(u)  InputArgumentSpecifications=<Enter example>  OutputArgumentSpecifications=<Enter example>
  Function Caller2 : FunctionCaller  FunctionPrototype=SCI_A_Transmit_one_shot_Suffix()  InputArgumentSpecifications=<Enter example>  OutputArgumentSpecifications=<Enter example>
  wires:
  Data Store Read/1 -> Function Caller1/1

== system CLA_Sample/Calibration,RMS, Fault Protection @5kHz/Calibration/Calibration_3phase ==
  function : TriggerPort  TriggerType=function-call  VariantControl=(inherit)
  Chart : Stateflow chart  TreatAsAtomicUnit=on
  Constant : Constant
  Data Store Read1 : DataStoreRead  DataStoreName=Calibration_Done_Phase_A  IndexOptions=Index vector (dialog)  Indices=1  OutputSizes=1
  Data Store Read2 : DataStoreRead  DataStoreName=Calibration_Done_Phase_B  IndexOptions=Index vector (dialog)  Indices=1  OutputSizes=1
  Data Store Read4 : DataStoreRead  DataStoreName=Calibration_Done_Phase_C  IndexOptions=Index vector (dialog)  Indices=1  OutputSizes=1
  Data Store Write : DataStoreWrite  DataStoreName=Calibration_Done  IndexOptions=Index vector (dialog)  Indices=1  OutputSizes=1
  wires:
  Chart/1(Calibration_Done) -> Data Store Write/1
  Data Store Read1/1 -> Chart/1(Calibration_Done_Phase_A)
  Constant/1 -> Chart/3(Calibration_Done_Phase_C), Chart/2(Calibration_Done_Phase_B)

== system CLA_Sample/Calibration,RMS, Fault Protection @5kHz/Calibration/Calibration_Phase_A ==
  function : TriggerPort  TriggerType=function-call  VariantControl=(inherit)
  Chart1 : Stateflow chart  TreatAsAtomicUnit=on
  Constant1 : Constant  Value=10000
  Data Store Read4 : DataStoreRead  DataStoreName=Inductor_Current_ADC_Phase_A  IndexOptions=Index vector (dialog)  Indices=1  OutputSizes=1
  Data Store Read5 : DataStoreRead  DataStoreName=Calibration_Done_Phase_A  IndexOptions=Index vector (dialog)  Indices=1  OutputSizes=1
  Data Store Read6 : DataStoreRead  DataStoreName=Vin_ADC_Phase_A  IndexOptions=Index vector (dialog)  Indices=1  OutputSizes=1
  Data Store Write4 : DataStoreWrite  DataStoreName=Calibration_Done_Phase_A  IndexOptions=Index vector (dialog)  Indices=1  OutputSizes=1
  Data Store Write5 : DataStoreWrite  DataStoreName=Inductor_Current_1_65_ADC_Phase_A  IndexOptions=Index vector (dialog)  Indices=1  OutputSizes=1
  Data Store Write6 : DataStoreWrite  DataStoreName=Vin_1_65_ADC_Phase_A  IndexOptions=Index vector (dialog)  Indices=1  OutputSizes=1
  wires:
  Chart1/1(output_signal_1) -> Data Store Write5/1
  Chart1/2(output_signal_2) -> Data Store Write6/1
  Constant1/1 -> Chart1/4(Counter_for_calibration)
  Data Store Read5/1 -> Chart1/1("Calibration_Done ")
  Chart1/3(Calibration_Done) -> Data Store Write4/1
  Data Store Read6/1 -> Chart1/3(input_signal_2)
  Data Store Read4/1 -> Chart1/2(input_signal_1)

== system CLA_Sample/Calibration,RMS, Fault Protection @5kHz/Calibration/Calibration_Phase_B ==
  function : TriggerPort  TriggerType=function-call  VariantControl=(inherit)
  Chart1 : Stateflow chart  TreatAsAtomicUnit=on
  Constant1 : Constant  Value=10000
  Data Store Read4 : DataStoreRead  DataStoreName=Inductor_Current_ADC_Phase_B  IndexOptions=Index vector (dialog)  Indices=1  OutputSizes=1
  Data Store Read5 : DataStoreRead  DataStoreName=Calibration_Done_Phase_B  IndexOptions=Index vector (dialog)  Indices=1  OutputSizes=1
  Data Store Read6 : DataStoreRead  DataStoreName=Vin_ADC_Phase_B  IndexOptions=Index vector (dialog)  Indices=1  OutputSizes=1
  Data Store Write4 : DataStoreWrite  DataStoreName=Calibration_Done_Phase_B  IndexOptions=Index vector (dialog)  Indices=1  OutputSizes=1
  Data Store Write5 : DataStoreWrite  DataStoreName=Inductor_Current_1_65_ADC_Phase_B  IndexOptions=Index vector (dialog)  Indices=1  OutputSizes=1
  Data Store Write6 : DataStoreWrite  DataStoreName=Vin_1_65_ADC_Phase_B  IndexOptions=Index vector (dialog)  Indices=1  OutputSizes=1
  wires:
  Chart1/1(output_signal_1) -> Data Store Write5/1
  Chart1/2(output_signal_2) -> Data Store Write6/1
  Constant1/1 -> Chart1/4(Counter_for_calibration)
  Data Store Read5/1 -> Chart1/1("Calibration_Done ")
  Chart1/3(Calibration_Done) -> Data Store Write4/1
  Data Store Read6/1 -> Chart1/3(input_signal_2)
  Data Store Read4/1 -> Chart1/2(input_signal_1)

== system CLA_Sample/Calibration,RMS, Fault Protection @5kHz/Calibration/Calibration_Phase_C ==
  function : TriggerPort  TriggerType=function-call  VariantControl=(inherit)
  Chart1 : Stateflow chart  TreatAsAtomicUnit=on
  Constant1 : Constant  Value=10000
  Data Store Read4 : DataStoreRead  DataStoreName=Inductor_Current_ADC_Phase_C  IndexOptions=Index vector (dialog)  Indices=1  OutputSizes=1
  Data Store Read5 : DataStoreRead  DataStoreName=Calibration_Done_Phase_C  IndexOptions=Index vector (dialog)  Indices=1  OutputSizes=1
  Data Store Read6 : DataStoreRead  DataStoreName=Vin_ADC_Phase_C  IndexOptions=Index vector (dialog)  Indices=1  OutputSizes=1
  Data Store Write4 : DataStoreWrite  DataStoreName=Calibration_Done_Phase_C  IndexOptions=Index vector (dialog)  Indices=1  OutputSizes=1
  Data Store Write5 : DataStoreWrite  DataStoreName=Inductor_Current_1_65_ADC_Phase_C  IndexOptions=Index vector (dialog)  Indices=1  OutputSizes=1
  Data Store Write6 : DataStoreWrite  DataStoreName=Vin_1_65_ADC_Phase_C  IndexOptions=Index vector (dialog)  Indices=1  OutputSizes=1
  wires:
  Chart1/1(output_signal_1) -> Data Store Write5/1
  Chart1/2(output_signal_2) -> Data Store Write6/1
  Constant1/1 -> Chart1/4(Counter_for_calibration)
  Data Store Read5/1 -> Chart1/1("Calibration_Done ")
  Chart1/3(Calibration_Done) -> Data Store Write4/1
  Data Store Read6/1 -> Chart1/3(input_signal_2)
  Data Store Read4/1 -> Chart1/2(input_signal_1)

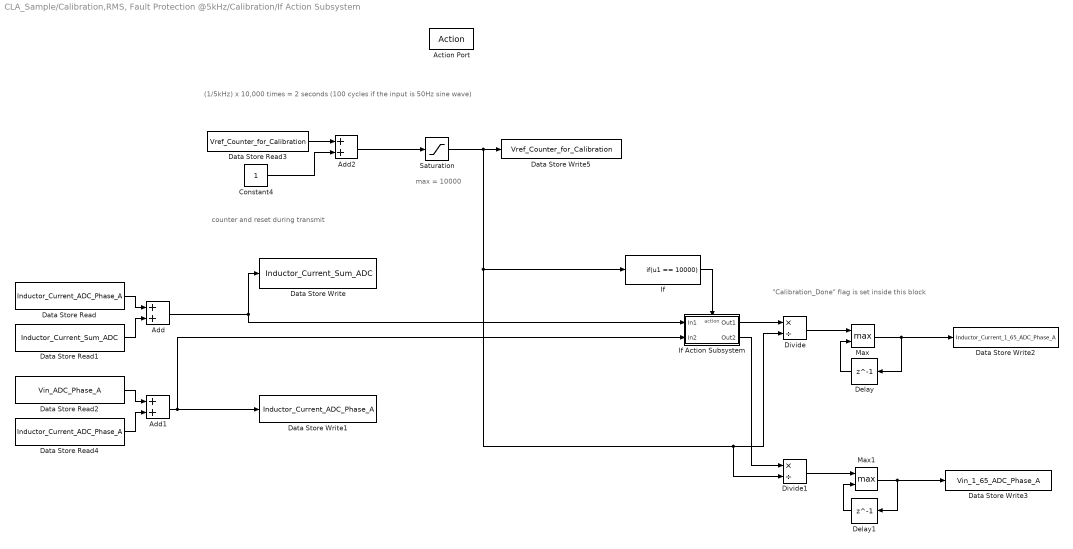
== system CLA_Sample/Calibration,RMS, Fault Protection @5kHz/Calibration/If Action Subsystem ==
  note: (1/5kHz) x 10,000 times = 2 seconds (100 cycles if the input is 50Hz sine wave)
  note: max = 10000
  note: counter and reset during transmit
  note: "Calibration_Done" flag is set inside this block
  Action Port : ActionPort
  Add : Sum
  Add1 : Sum
  Add2 : Sum
  Constant4 : Constant
  Data Store Read : DataStoreRead  DataStoreName=Inductor_Current_ADC_Phase_A  IndexOptions=Index vector (dialog)  Indices=1  OutputSizes=1
  Data Store Read1 : DataStoreRead  DataStoreName=Inductor_Current_Sum_ADC  IndexOptions=Index vector (dialog)  Indices=1  OutputSizes=1
  Data Store Read2 : DataStoreRead  DataStoreName=Vin_ADC_Phase_A  IndexOptions=Index vector (dialog)  Indices=1  OutputSizes=1
  Data Store Read3 : DataStoreRead  DataStoreName=Vref_Counter_for_Calibration  IndexOptions=Index vector (dialog)  Indices=1  OutputSizes=1
  Data Store Read4 : DataStoreRead  DataStoreName=Inductor_Current_ADC_Phase_A  IndexOptions=Index vector (dialog)  Indices=1  OutputSizes=1
  Data Store Write : DataStoreWrite  DataStoreName=Inductor_Current_Sum_ADC  IndexOptions=Index vector (dialog)  Indices=1  OutputSizes=1
  Data Store Write1 : DataStoreWrite  DataStoreName=Inductor_Current_ADC_Phase_A  IndexOptions=Index vector (dialog)  Indices=1  OutputSizes=1
  Data Store Write2 : DataStoreWrite  DataStoreName=Inductor_Current_1_65_ADC_Phase_A  IndexOptions=Index vector (dialog)  Indices=1  OutputSizes=1
  Data Store Write3 : DataStoreWrite  DataStoreName=Vin_1_65_ADC_Phase_A  IndexOptions=Index vector (dialog)  Indices=1  OutputSizes=1
  Data Store Write5 : DataStoreWrite  DataStoreName=Vref_Counter_for_Calibration  IndexOptions=Index vector (dialog)  Indices=1  OutputSizes=1
  Delay : Delay  DelayLength=1
  Delay1 : Delay  DelayLength=1
  Divide : Product  Inputs=*/
  Divide1 : Product  Inputs=*/
  If : If  IfExpression=u1 == 10000  ShowElse=off
  If Action Subsystem : Subsystem  TreatAsAtomicUnit=on
  Max : MinMax  Function=max  Inputs=2
  Max1 : MinMax  Function=max  Inputs=2
  Saturation : Saturate  UpperLimit=10001  LowerLimit=0
  wires:
  Max1/1 -> Data Store Write3/1, Delay1/1
  Saturation/1 -> Data Store Write5/1, Divide/2, Divide1/2, If/1
  Delay/1 -> Max/2
  If/1 -> If Action Subsystem/Action
  Delay1/1 -> Max1/2
  Data Store Read2/1 -> Add1/1
  Data Store Read4/1 -> Add1/2
  Add/1 -> If Action Subsystem/1(In1), Data Store Write/1
  Data Store Read/1 -> Add/1
  Constant4/1 -> Add2/2
  Data Store Read3/1 -> Add2/1
  Add2/1 -> Saturation/1
  Data Store Read1/1 -> Add/2
  Max/1 -> Data Store Write2/1, Delay/1
  Add1/1 -> If Action Subsystem/2(In2), Data Store Write1/1
  If Action Subsystem/1(Out1) -> Divide/1
  Divide/1 -> Max/1
  If Action Subsystem/2(Out2) -> Divide1/1
  Divide1/1 -> Max1/1
